simulink model "BCM_TopLevelModel"  (R2025b)
settings: Solver=VariableStepAuto  StartTime=0.0  StopTime=10.0  RelTol=1e-3
settings Model: Creator=Sai Krishna  LastModifiedBy=Sai Krishna

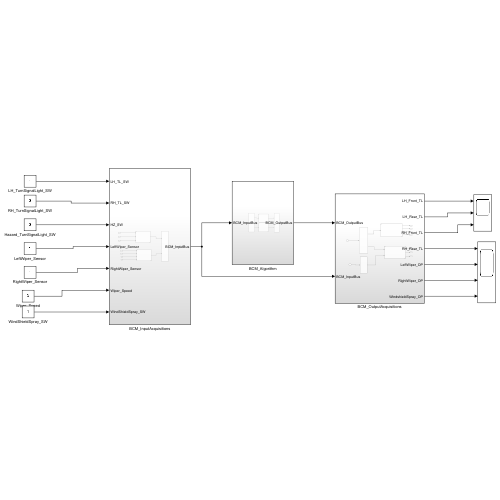
[thumbnail: Simulink's stored preview of the top-level diagram]
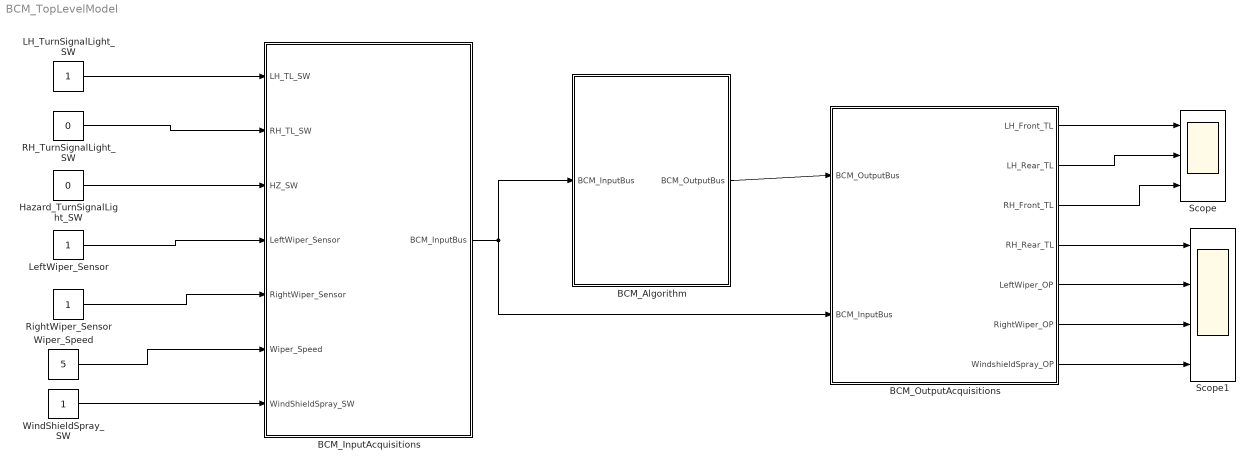
== system BCM_TopLevelModel ==
  BCM_Algorithm : Subsystem
  BCM_InputAcquisitions : Subsystem
  BCM_OutputAcquisitions : Subsystem
  "Hazard_TurnSignalLight_SW " : Constant  Value=0  OutDataTypeStr=boolean
  "LH_TurnSignalLight_SW " : Constant  OutDataTypeStr=boolean
  LeftWiper_Sensor : Constant  OutDataTypeStr=boolean
  "RH_TurnSignalLight_SW " : Constant  Value=0  OutDataTypeStr=boolean
  RightWiper_Sensor : Constant  OutDataTypeStr=boolean
  Scope : Scope  NumInputPorts=3
  Scope1 : Scope  NumInputPorts=4
  WindShieldSpray_SW : Constant  OutDataTypeStr=boolean
  Wiper_Speed : Constant  Value=5  OutDataTypeStr=double
  wires:
  BCM_InputAcquisitions/1(BCM_InputBus) -> BCM_Algorithm/1(BCM_InputBus), BCM_OutputAcquisitions/2(BCM_InputBus)
  BCM_Algorithm/1(BCM_OutputBus) -> BCM_OutputAcquisitions/1(BCM_OutputBus)
  "Hazard_TurnSignalLight_SW "/1 -> BCM_InputAcquisitions/3(HZ_SW)
  "LH_TurnSignalLight_SW "/1 -> BCM_InputAcquisitions/1(LH_TL_SW)
  "RH_TurnSignalLight_SW "/1 -> BCM_InputAcquisitions/2(RH_TL_SW)
  Wiper_Speed/1 -> BCM_InputAcquisitions/6(Wiper_Speed)
  RightWiper_Sensor/1 -> BCM_InputAcquisitions/5(RightWiper_Sensor)
  LeftWiper_Sensor/1 -> BCM_InputAcquisitions/4(LeftWiper_Sensor)
  WindShieldSpray_SW/1 -> BCM_InputAcquisitions/7(WindShieldSpray_SW)
  BCM_OutputAcquisitions/1(LH_Front_TL) -> Scope/1
  BCM_OutputAcquisitions/2(LH_Rear_TL) -> Scope/2
  BCM_OutputAcquisitions/3(RH_Front_TL) -> Scope/3
  BCM_OutputAcquisitions/4(RH_Rear_TL) -> Scope1/1
  BCM_OutputAcquisitions/5(LeftWiper_OP) -> Scope1/2
  BCM_OutputAcquisitions/6(RightWiper_OP) -> Scope1/3
  BCM_OutputAcquisitions/7(WindshieldSpray_OP) -> Scope1/4

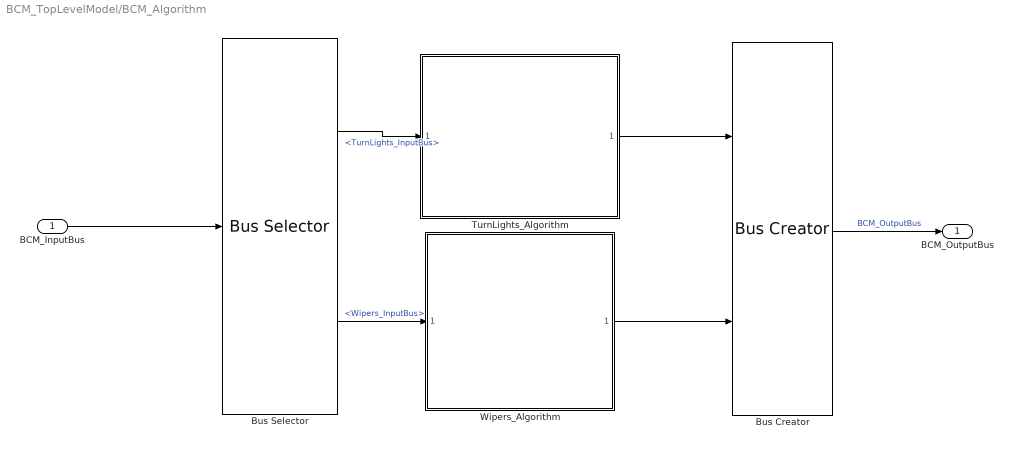
== system BCM_TopLevelModel/BCM_Algorithm ==
  BCM_InputBus : Inport  OutDataTypeStr=Bus: BCM_InputBus
  Bus Creator : BusCreator  Inputs=2  OutDataTypeStr=Bus: BCM_OutputBus
      settings: InheritFromInputs=off
  Bus Selector : BusSelector  OutputSignals=TurnLights_InputBus,Wipers_InputBus
  TurnLights_Algorithm : Subsystem  ReferencedSubsystem=TurnLights_Algorithm
  Wipers_Algorithm : Subsystem  ReferencedSubsystem=Wipers_Algorithm
  BCM_OutputBus : Outport  OutDataTypeStr=Bus: BCM_OutputBus
  wires:
  BCM_InputBus/1 -> Bus Selector/1
  Bus Selector/1 -> TurnLights_Algorithm/1  "<TurnLights_InputBus>"
  Bus Selector/2 -> Wipers_Algorithm/1  "<Wipers_InputBus>"
  TurnLights_Algorithm/1 -> Bus Creator/1
  Wipers_Algorithm/1 -> Bus Creator/2
  Bus Creator/1 -> BCM_OutputBus/1  "BCM_OutputBus"

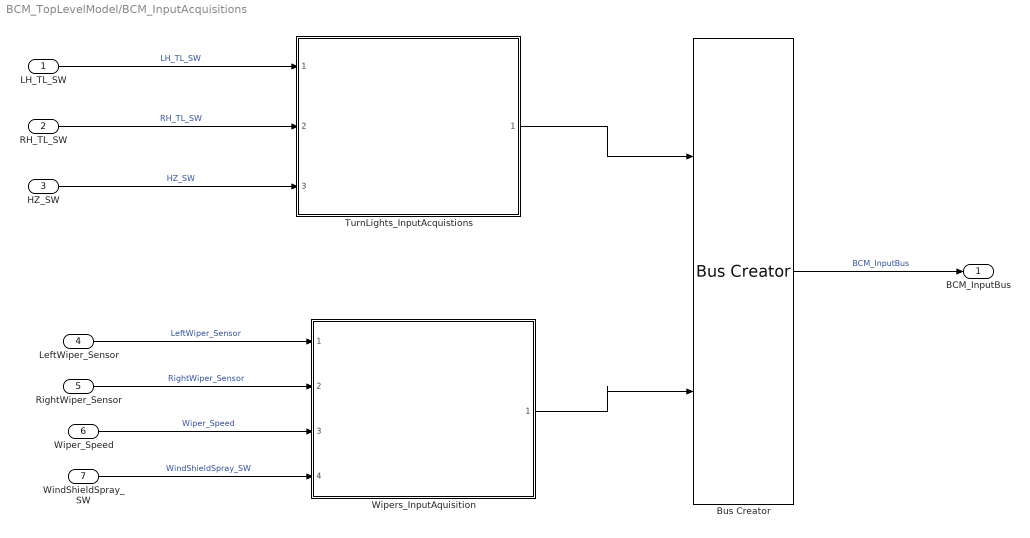
== system BCM_TopLevelModel/BCM_InputAcquisitions ==
  LH_TL_SW : Inport  OutDataTypeStr=boolean
  RH_TL_SW : Inport  Port=2  OutDataTypeStr=boolean
  HZ_SW : Inport  Port=3  OutDataTypeStr=boolean
  LeftWiper_Sensor : Inport  Port=4  OutDataTypeStr=boolean
  RightWiper_Sensor : Inport  Port=5  OutDataTypeStr=boolean
  Wiper_Speed : Inport  Port=6  OutDataTypeStr=double
  WindShieldSpray_SW : Inport  Port=7  OutDataTypeStr=boolean
  Bus Creator : BusCreator  Inputs=2  OutDataTypeStr=Bus: BCM_InputBus
      settings: InheritFromInputs=off
  TurnLights_InputAcquistions : Subsystem  ReferencedSubsystem=TurnLights_InputAcquistions
  Wipers_InputAquisition : Subsystem  ReferencedSubsystem=Wipers_InputAquisition
  BCM_InputBus : Outport  OutDataTypeStr=Bus: BCM_InputBus
  wires:
  LH_TL_SW/1 -> TurnLights_InputAcquistions/1  "LH_TL_SW"
  HZ_SW/1 -> TurnLights_InputAcquistions/3  "HZ_SW"
  RH_TL_SW/1 -> TurnLights_InputAcquistions/2  "RH_TL_SW"
  Wiper_Speed/1 -> Wipers_InputAquisition/3  "Wiper_Speed"
  RightWiper_Sensor/1 -> Wipers_InputAquisition/2  "RightWiper_Sensor"
  WindShieldSpray_SW/1 -> Wipers_InputAquisition/4  "WindShieldSpray_SW"
  LeftWiper_Sensor/1 -> Wipers_InputAquisition/1  "LeftWiper_Sensor"
  TurnLights_InputAcquistions/1 -> Bus Creator/1
  Wipers_InputAquisition/1 -> Bus Creator/2
  Bus Creator/1 -> BCM_InputBus/1  "BCM_InputBus"

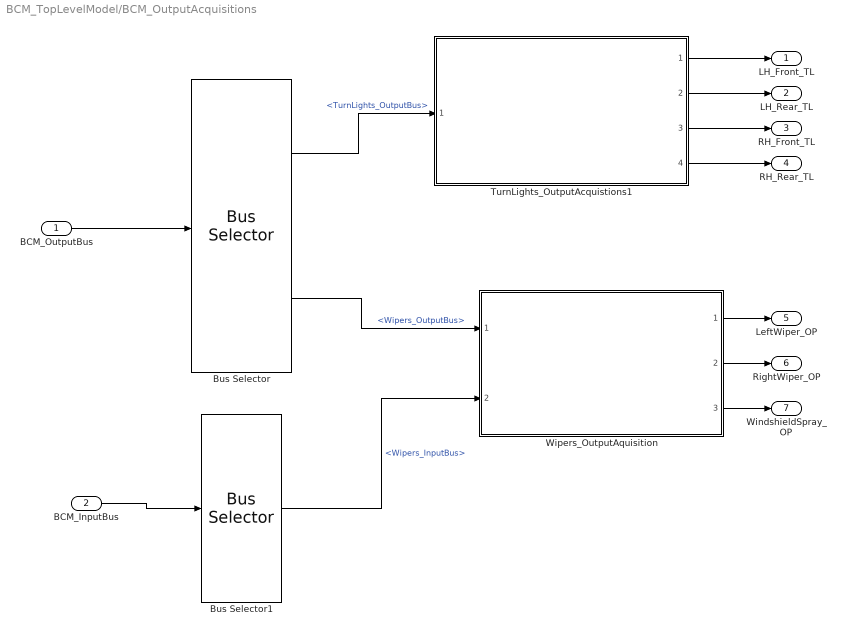
== system BCM_TopLevelModel/BCM_OutputAcquisitions ==
  BCM_OutputBus : Inport  OutDataTypeStr=Bus: BCM_OutputBus
  BCM_InputBus : Inport  Port=2
  Bus Selector : BusSelector  OutputSignals=TurnLights_OutputBus,Wipers_OutputBus
  Bus Selector1 : BusSelector  OutputSignals=Wipers_InputBus
  TurnLights_OutputAcquistions1 : Subsystem  ReferencedSubsystem=TurnLights_OutputAcquistions1
  Wipers_OutputAquisition : Subsystem  ReferencedSubsystem=Wipers_OutputAquisition
  LH_Front_TL : Outport
  LH_Rear_TL : Outport  Port=2
  RH_Front_TL : Outport  Port=3
  RH_Rear_TL : Outport  Port=4
  LeftWiper_OP : Outport  Port=5  OutDataTypeStr=double
  RightWiper_OP : Outport  Port=6  OutDataTypeStr=double
  WindshieldSpray_OP : Outport  Port=7  OutDataTypeStr=double
  wires:
  BCM_OutputBus/1 -> Bus Selector/1
  Bus Selector/2 -> Wipers_OutputAquisition/1  "<Wipers_OutputBus>"
  Bus Selector/1 -> TurnLights_OutputAcquistions1/1  "<TurnLights_OutputBus>"
  TurnLights_OutputAcquistions1/2 -> LH_Rear_TL/1
  TurnLights_OutputAcquistions1/3 -> RH_Front_TL/1
  TurnLights_OutputAcquistions1/4 -> RH_Rear_TL/1
  TurnLights_OutputAcquistions1/1 -> LH_Front_TL/1
  Wipers_OutputAquisition/3 -> WindshieldSpray_OP/1
  Wipers_OutputAquisition/2 -> RightWiper_OP/1
  Wipers_OutputAquisition/1 -> LeftWiper_OP/1
  BCM_InputBus/1 -> Bus Selector1/1
  Bus Selector1/1 -> Wipers_OutputAquisition/2  "<Wipers_InputBus>"
